simulink model "P5"  (R2025a)
settings: Solver=VariableStepAuto  StartTime=0.0  StopTime=10.0  RelTol=1e-3
values from neighbouring files (symbols this model uses):
  Cf = [0.05 0 ; 0 0]    [Params.m]
  fd = [10 0]    [Params.m]
  K = [1000 0 ; 0 0]    [Params.m]
  Kd = [5000 0 ; 0 5000]    [Params.m]
  Kf = [0.03 0 ; 0 0]    [Params.m]
  Kp = [5000 0 ; 0 5000]    [Params.m]
  Md = [1000 0 ; 0 1000]    [Params.m]
  Xr = [1.2 0.7]    [Params.m]
settings Model: Creator=Chenfu  LastModifiedBy=Chenfu

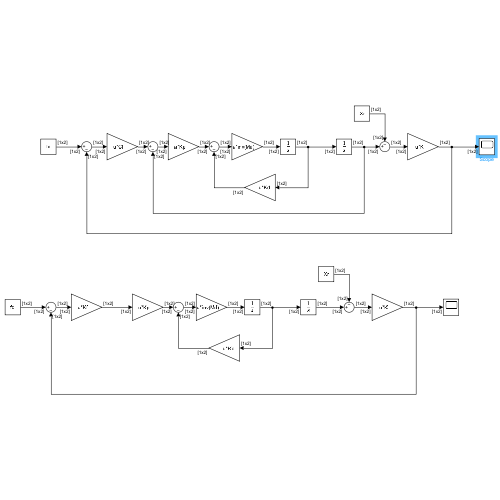
[thumbnail: Simulink's stored preview of the top-level diagram]
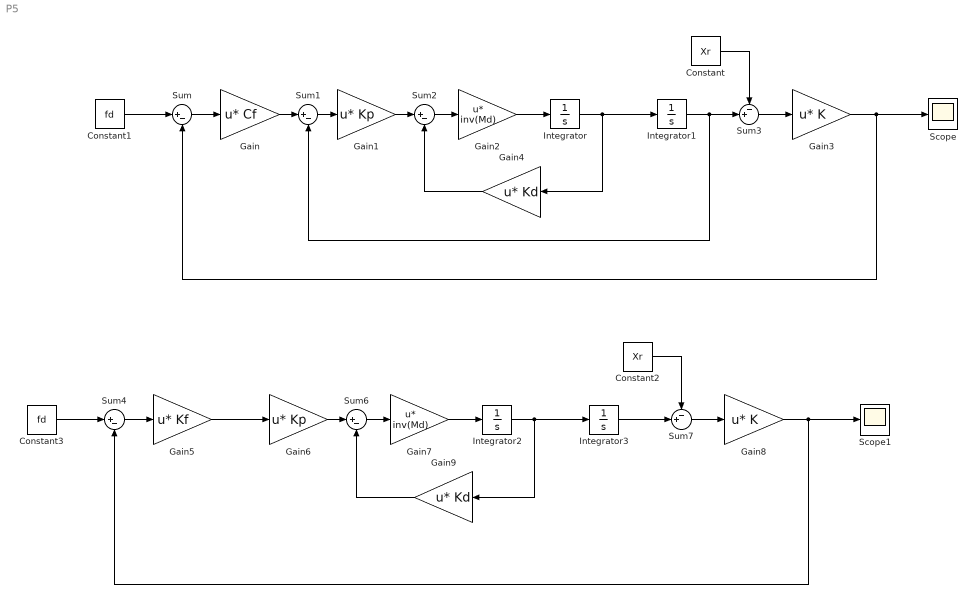
== system P5 ==
  Constant : Constant  Value=Xr  VectorParams1D=off
  Constant1 : Constant  Value=fd  VectorParams1D=off
  Constant2 : Constant  Value=Xr  VectorParams1D=off
  Constant3 : Constant  Value=fd  VectorParams1D=off
  Gain : Gain  Gain=Cf  Multiplication=Matrix(u*K)
  Gain1 : Gain  Gain=Kp  Multiplication=Matrix(u*K)
  Gain2 : Gain  Gain=inv(Md)  Multiplication=Matrix(u*K)
  Gain3 : Gain  Gain=K  Multiplication=Matrix(u*K)
  Gain4 : Gain  Gain=Kd  Multiplication=Matrix(u*K)
  Gain5 : Gain  Gain=Kf  Multiplication=Matrix(u*K)
  Gain6 : Gain  Gain=Kp  Multiplication=Matrix(u*K)
  Gain7 : Gain  Gain=inv(Md)  Multiplication=Matrix(u*K)
  Gain8 : Gain  Gain=K  Multiplication=Matrix(u*K)
  Gain9 : Gain  Gain=Kd  Multiplication=Matrix(u*K)
  Integrator{,1..3} (4 alike) : Integrator
  Scope : Scope
      settings: ActiveDisplayYMinimum=-51.357002526142537  ActiveDisplayYMaximum=21.37445623431444
  Scope1 : Scope
      settings: ActiveDisplayYMinimum=-114.17435624009036  ActiveDisplayYMaximum=78.172057626050076
  Sum{,1..2,4,6} (5 alike) : Sum  Inputs=|+-
  Sum3 : Sum  Inputs=-+|
  Sum7 : Sum  Inputs=-+|
  wires:
  Gain2/1 -> Integrator/1
  Sum/1 -> Gain/1
  Gain/1 -> Sum1/1
  Sum1/1 -> Gain1/1
  Gain1/1 -> Sum2/1
  Sum2/1 -> Gain2/1
  Integrator/1 -> Integrator1/1, Gain4/1
  Integrator1/1 -> Sum3/2, Sum1/2
  Sum3/1 -> Gain3/1
  Gain3/1 -> Sum/2, Scope/1
  Gain4/1 -> Sum2/2
  Constant/1 -> Sum3/1
  Constant1/1 -> Sum/1
  Constant2/1 -> Sum7/1
  Constant3/1 -> Sum4/1
  Sum6/1 -> Gain7/1
  Sum4/1 -> Gain5/1
  Gain8/1 -> Sum4/2, Scope1/1
  Sum7/1 -> Gain8/1
  Integrator2/1 -> Integrator3/1, Gain9/1
  Integrator3/1 -> Sum7/2
  Gain9/1 -> Sum6/2
  Gain5/1 -> Gain6/1
  Gain6/1 -> Sum6/1
  Gain7/1 -> Integrator2/1
